simulink model "balancer"  (R2020a)
settings: Solver=FixedStepDiscrete  StartTime=0.0  StopTime=inf  FixedStep=0.03  RelTol=1e-3  EnableMultiTasking=on
values from neighbouring files (symbols this model uses):
  K = lqr(A, B, Q, R)    [lab06.m]
  Rw = 0.0216    [balance_ode.m]    (also in lab06.m)
undefined symbols (not defined in the file or in its folder): DiscIntNeverNeededParam
libraries: MinSegLibrary_M1V4 x2, simulink x1
settings Model: SimulationMode=external  SILPILModeSetting=veronly  ExtModeTrigDuration=2  Creator=Alec  LastModifiedBy=donelp
settings DataIOCC: LimitDataPoints=on  SaveFormat=Array  ReturnWorkspaceOutputs=off
settings OptimizationCC: EnhancedBackFolding=on  PassReuseOutputArgsAs=Individual arguments  ExpressionDepthLimit=2147483647  ZeroExternalMemoryAtStartup=off  ZeroInternalMemoryAtStartup=off  MaxStackSize=64  OptimizeBlockOrder=speed  DifferentSizesBufferReuse=on  OptimizationCustomize=off  EfficientTunableParamExpr=on
settings DebuggingCC: UnderspecifiedInitializationDetection=Classic  MergeDetectMultiDrivingBlocksExec=none  ParameterTunabilityLossMsg=error  StateNameClashWarn=warning  SFUnexpectedBacktrackingDiag=warning  SFNoUnconditionalDefaultTransitionDiag=warning  SFExecutionAtInitializationDiag=none  ArithmeticOperatorsInVariantConditions=warning
settings HardwareCC: ProdBitPerInt=16  ProdBitPerPointer=16  ProdBitPerSizeT=16  ProdBitPerPtrDiffT=16  ProdLargestAtomicFloat=None  ProdWordSize=8  ProdHWDeviceType=Atmel->AVR  UseEmbeddedCoderFeatures=off  UseSimulinkCoderFeatures=off
settings ModelReferenceCC: PropagateSignalLabelsOutOfModel=off
settings SFSimCC: SimUseLocalCustomCode=off  MATLABDynamicMemAlloc=off  CustomCodeUndefinedFunction=UseInterfaceOnly
settings RTWCC: SystemTargetFile=ert.tlc  HardwareBoard=Arduino Mega 2560  TLCOptions=-aInlineSetEventsForThisBaseRateFcn=TLC_FALSE -aSuppressMultiTaskScheduler=TLC_FALSE -aRateBasedStepFcn=1  TemplateMakefile=ert_default_tmf  RTWVerbose=off  RTWUseLocalCustomCode=off  Toolchain=Arduino AVR  BuildConfiguration=Faster Runs
settings CodeAppCC: ForceParamTrailComments=on  IgnoreCustomStorageClasses=off  OperatorAnnotations=on  SimulinkDataObjDesc=on  SFDataObjDesc=on  MangleLength=10  CustomSymbolStrType=$N$R$M  InsertBlockDesc=on  InternalIdentifier=Classic
settings ERTTargetCC: SupportContinuousTime=on  SupportNonInlinedSFcns=on  SupportVariableSizeSignals=on  ExtModeStaticAllocSize=2048
settings ConfigComp: CovMetricSettings=dw  CovHtmlReporting=on  CovSaveCumulativeToWorkspaceVar=on  CovSaveSingleToWorkspaceVar=on  CovExternalEMLEnable=off

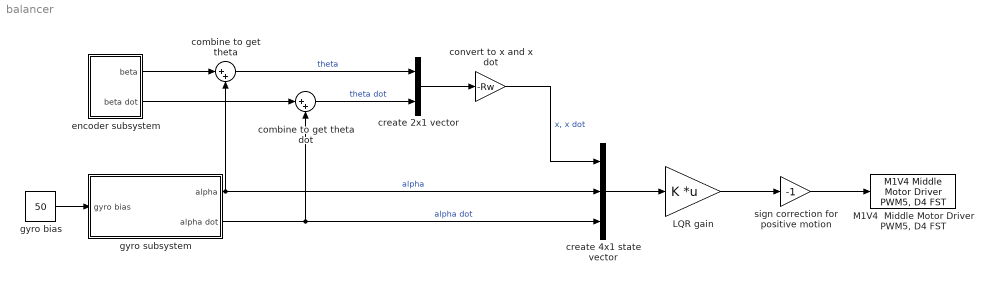
== system balancer ==
  LQR gain : Gain  Gain=K  Multiplication=Matrix(K*u)
  "M1V4  Middle Motor Driver PWM5, D4 FST" : MinSegLibrary_M1V4/M1V4  Middle Motor Driver PWM5, D4 FST  Vsupply=3.56
      settings: SourceProductName=Rensselaer Arduino Support Package
  combine to get theta : Sum  Inputs=|++
  combine to get theta dot : Sum  Inputs=|++
  convert to x and x dot : Gain  Gain=-Rw
  create 2x1 vector : Mux  Inputs=2
  create 4x1 state vector : Mux  Inputs=3
  encoder subsystem : Subsystem
  gyro bias : Constant  Value=50
  gyro subsystem : Subsystem
  sign correction for positive motion : Gain  Gain=-1
  wires:
  gyro subsystem/2(alpha dot) -> create 4x1 state vector/3, combine to get theta dot/2  "alpha dot"
  gyro subsystem/1(alpha) -> create 4x1 state vector/2, combine to get theta/2  "alpha"
  encoder subsystem/1(beta) -> combine to get theta/1
  encoder subsystem/2(beta dot) -> combine to get theta dot/1
  combine to get theta/1 -> create 2x1 vector/1  "theta"
  combine to get theta dot/1 -> create 2x1 vector/2  "theta dot"
  create 2x1 vector/1 -> convert to x and x dot/1
  convert to x and x dot/1 -> create 4x1 state vector/1  "x, x dot"
  gyro bias/1 -> gyro subsystem/1(gyro bias)
  create 4x1 state vector/1 -> LQR gain/1
  LQR gain/1 -> sign correction for positive motion/1
  sign correction for positive motion/1 -> "M1V4  Middle Motor Driver PWM5, D4 FST"/1

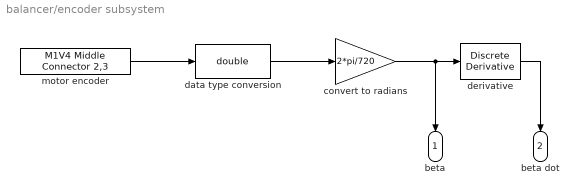
== system balancer/encoder subsystem ==
  convert to radians : Gain  Gain=2*pi/720
  data type conversion : DataTypeConversion  OutDataTypeStr=double
  derivative : simulink/Discrete/Discrete Derivative  gainval=1.0  ICPrevScaledInput=0.0  OutMin=[]  OutMax=[]  OutDataType=fixdt(1, 16)  OutScaling=2^-10  DoSatur=off
  motor encoder : MinSegLibrary_M1V4/M1V4 Middle Connector 2,3  Encoder=0  PinA=3  PinB=2
      settings: SourceProductName=Rensselaer Arduino Support Package
  beta : Outport
  beta dot : Outport  Port=2
  wires:
  convert to radians/1 -> beta/1, derivative/1
  data type conversion/1 -> convert to radians/1
  derivative/1 -> beta dot/1
  motor encoder/1 -> data type conversion/1

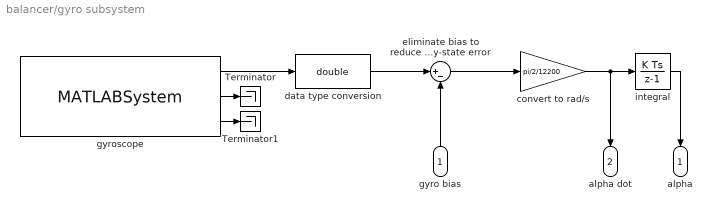
== system balancer/gyro subsystem ==
  gyro bias : Inport
  Terminator : Terminator
  Terminator1 : Terminator
  convert to rad/s : Gain  Gain=pi/2/12200
  data type conversion : DataTypeConversion  OutDataTypeStr=double
  eliminate bias to reduce steady-state error : Sum  Inputs=|+-
  gyroscope : MATLABSystem  System=soMPU6050Gyro  DLPFmode=0
      mask Type: soMPU6050Gyro
      mask Display:
      | disp('soMPU6050Gyro');
      | port_label('output',1,'xvel');
      | port_label('output',2,'yvel');
      | port_label('output',3,'zvel');
  integral : DiscreteIntegrator  SampleTime=-1  ICPrevOutput=DiscIntNeverNeededParam  ICPrevScaledInput=DiscIntNeverNeededParam
  alpha : Outport
  alpha dot : Outport  Port=2
  wires:
  gyroscope/1 -> data type conversion/1
  convert to rad/s/1 -> alpha dot/1, integral/1
  gyro bias/1 -> eliminate bias to reduce steady-state error/2
  gyroscope/3 -> Terminator1/1
  gyroscope/2 -> Terminator/1
  eliminate bias to reduce steady-state error/1 -> convert to rad/s/1
  integral/1 -> alpha/1
  data type conversion/1 -> eliminate bias to reduce steady-state error/1
